simulink model "linearTFDescentralizado_NaoMinimo"  (Simulink 7.7)
settings: Solver=ode45  StartTime=0.0  StopTime=1900  RelTol=1e-3
values from neighbouring files (symbols this model uses):
  QT =     [FaseMinima.mat]    (also in FaseNaoMinima.mat; FaseNaoMinimaMudandoApenasGama.mat; settup.m = dynamics())
settings Model: Creator=Arthur  LastModifiedBy=Arthur

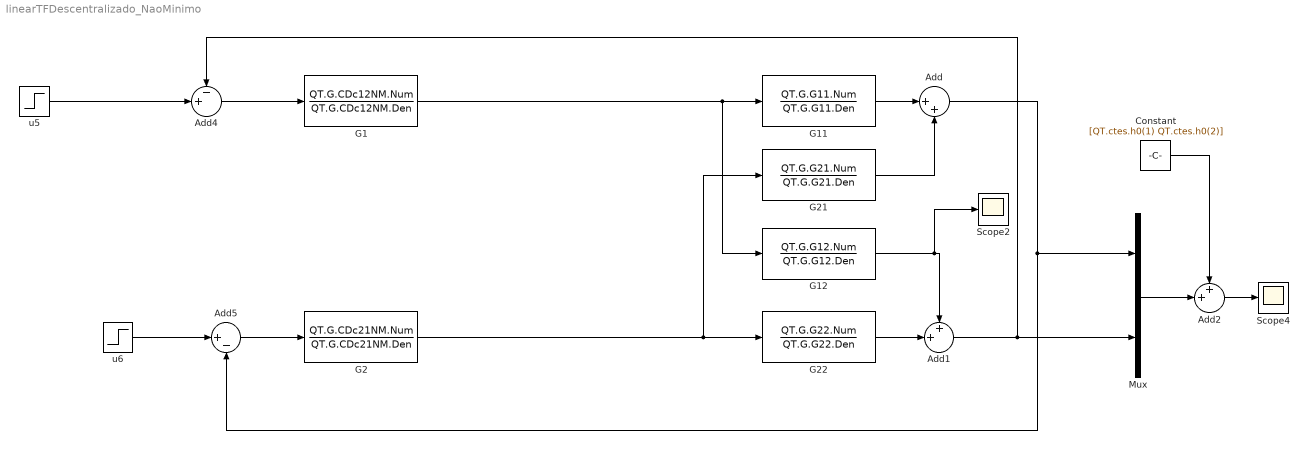
== system linearTFDescentralizado_NaoMinimo ==
  Add : Sum  Inputs=|++
  Add1 : Sum  Inputs=++|
  Add2 : Sum  Inputs=++|
  Add4 : Sum  Inputs=-+|
  Add5 : Sum  Inputs=|+-
  Constant : Constant  Value=[QT.ctes.h0(1) QT.ctes.h0(2)]
  G1 : TransferFcn  Numerator=QT.G.CDc12NM.Num  Denominator=QT.G.CDc12NM.Den
  G11 : TransferFcn  Numerator=QT.G.G11.Num  Denominator=QT.G.G11.Den
  G12 : TransferFcn  Numerator=QT.G.G12.Num  Denominator=QT.G.G12.Den
  G2 : TransferFcn  Numerator=QT.G.CDc21NM.Num  Denominator=QT.G.CDc21NM.Den
  G21 : TransferFcn  Numerator=QT.G.G21.Num  Denominator=QT.G.G21.Den
  G22 : TransferFcn  Numerator=QT.G.G22.Num  Denominator=QT.G.G22.Den
  Mux : Mux  Inputs=2
  Scope2 : Scope
      settings: TimeRange=10  SaveName=ScopeData2
  Scope4 : Scope
      settings: TimeRange=10  SaveName=Simulado
  u5 : Step  Time=1100  SampleTime=0
  u6 : Step  Time=300  SampleTime=0
  wires:
  Add/1 -> Mux/1, Add5/2
  Add1/1 -> Mux/2, Add4/1
  Add5/1 -> G2/1
  G21/1 -> Add/2
  Add4/1 -> G1/1
  G11/1 -> Add/1
  G22/1 -> Add1/2
  G12/1 -> Add1/1, Scope2/1
  G1/1 -> G12/1, G11/1
  G2/1 -> G21/1, G22/1
  Mux/1 -> Add2/2
  Add2/1 -> Scope4/1
  Constant/1 -> Add2/1
  u5/1 -> Add4/2
  u6/1 -> Add5/1
